simulink model "modelloTD_es1_sol2"  (R2021a)
settings: Solver=FixedStepDiscrete  StartTime=0.0  StopTime=10.0  FixedStep=0.001  RelTol=1e-3
values from neighbouring files (symbols this model uses):
  k = sym('k')    [fdt_es1.m]
  M1 = sym('M1')    [fdt_es1.m]
  M2 = sym('M2')    [fdt_es1.m]
undefined symbols (not defined in the file or in its folder): A1, A2, B1, B2, C1, C2
settings Model: Creator=User_LABORATORIO  LastModifiedBy=User_LABORATORIO

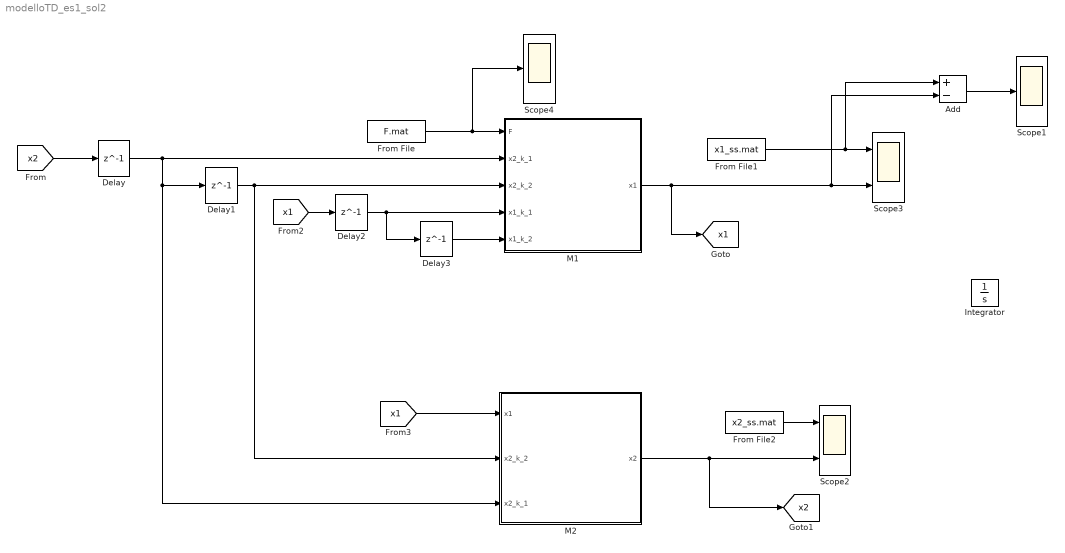
== system modelloTD_es1_sol2 ==
  Add : Sum  Inputs=+-
  Delay{,1..3} (4 alike) : Delay  DelayLength=1  InitialCondition=0
  From File : FromFile  FileName=F.mat  SampleTime=0
  From File1 : FromFile  FileName=x1_ss.mat  SampleTime=0
  From File2 : FromFile  FileName=x2_ss.mat  SampleTime=0
  Integrator : Integrator
  M1 : Subsystem
  M2 : Subsystem
  Scope1 : Scope
  Scope2 : Scope  NumInputPorts=2
  Scope3 : Scope  NumInputPorts=2
  Scope4 : Scope
  tag scope: x1=global, x2=global
  wires:
  Delay/1 -> M2/3(x2_k_1), Delay1/1, M1/2(x2_k_1)
  Add/1 -> Scope1/1
  M2/1(x2) -> [x2], Scope2/2
  [x1] -> M2/1(x1)
  From File1/1 -> Scope3/1, Add/1
  Delay3/1 -> M1/5(x1_k_2)
  [x1] -> Delay2/1
  Delay1/1 -> M2/2(x2_k_2), M1/3(x2_k_2)
  Delay2/1 -> Delay3/1, M1/4(x1_k_1)
  M1/1(x1) -> Scope3/2, Add/2, [x1]
  [x2] -> Delay/1
  From File/1 -> Scope4/1, M1/1(F)
  From File2/1 -> Scope2/1

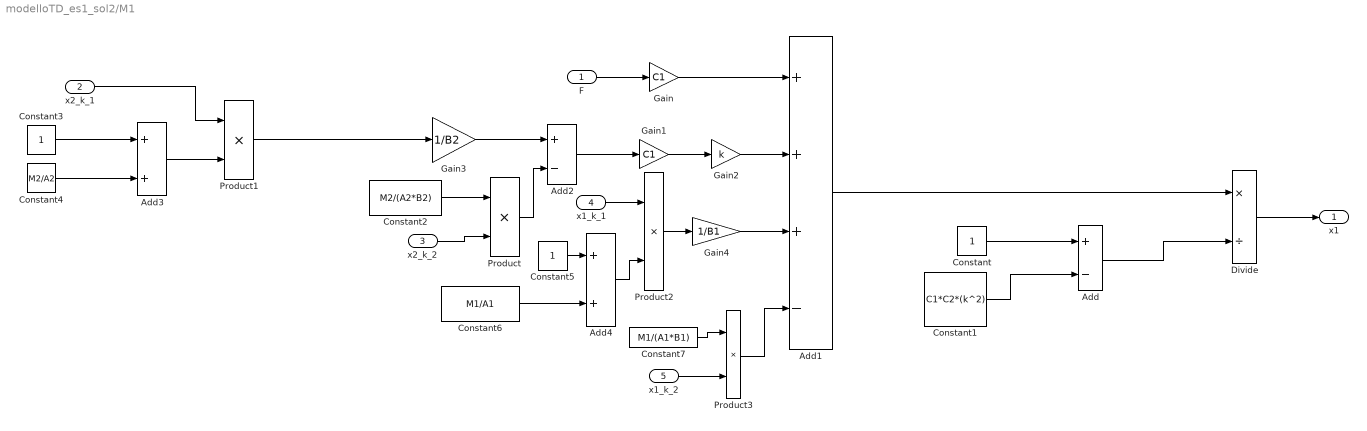
== system modelloTD_es1_sol2/M1 ==
  F : Inport
  x2_k_1 : Inport  Port=2
  x2_k_2 : Inport  Port=3
  x1_k_1 : Inport  Port=4
  x1_k_2 : Inport  Port=5
  Add : Sum  Inputs=+-
  Add1 : Sum  Inputs=+++-
  Add2 : Sum  Inputs=+-
  Add3 : Sum
  Add4 : Sum
  Constant : Constant
  Constant1 : Constant  Value=C1*C2*(k^2)
  Constant2 : Constant  Value=M2/(A2*B2)
  Constant3 : Constant
  Constant4 : Constant  Value=M2/A2
  Constant5 : Constant
  Constant6 : Constant  Value=M1/A1
  Constant7 : Constant  Value=M1/(A1*B1)
  Divide : Product  Inputs=*/
  Gain : Gain  Gain=C1
  Gain1 : Gain  Gain=C1
  Gain2 : Gain  Gain=k
  Gain3 : Gain  Gain=1/B2
  Gain4 : Gain  Gain=1/B1
  Product{,1..3} (4 alike) : Product
  x1 : Outport
  wires:
  Gain/1 -> Add1/1
  Constant3/1 -> Add3/1
  Product3/1 -> Add1/4
  Add/1 -> Divide/2
  Product/1 -> Add2/2
  x2_k_1/1 -> Product1/1
  F/1 -> Gain/1
  Constant/1 -> Add/1
  Divide/1 -> x1/1
  Constant1/1 -> Add/2
  Gain2/1 -> Add1/2
  Product1/1 -> Gain3/1
  Add1/1 -> Divide/1
  Constant4/1 -> Add3/2
  Gain1/1 -> Gain2/1
  Add3/1 -> Product1/2
  x1_k_2/1 -> Product3/2
  Add2/1 -> Gain1/1
  x2_k_2/1 -> Product/2
  Gain3/1 -> Add2/1
  x1_k_1/1 -> Product2/1
  Constant5/1 -> Add4/1
  Constant7/1 -> Product3/1
  Constant2/1 -> Product/1
  Add4/1 -> Product2/2
  Constant6/1 -> Add4/2
  Product2/1 -> Gain4/1
  Gain4/1 -> Add1/3

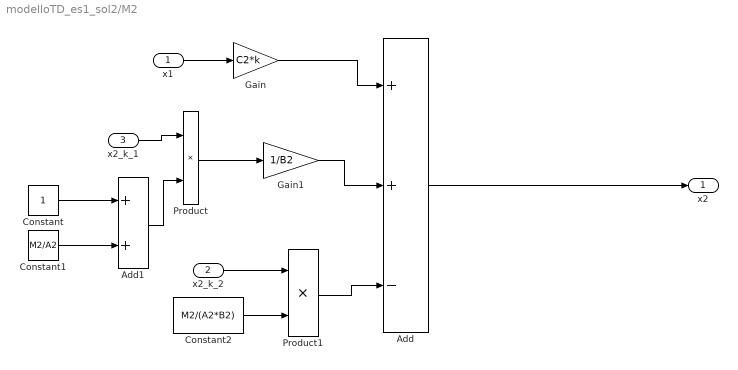
== system modelloTD_es1_sol2/M2 ==
  x1 : Inport
  x2_k_2 : Inport  Port=2
  x2_k_1 : Inport  Port=3
  Add : Sum  Inputs=++-
  Add1 : Sum
  Constant : Constant
  Constant1 : Constant  Value=M2/A2
  Constant2 : Constant  Value=M2/(A2*B2)
  Gain : Gain  Gain=C2*k
  Gain1 : Gain  Gain=1/B2
  Product : Product
  Product1 : Product
  x2 : Outport
  wires:
  Gain/1 -> Add/1
  Constant/1 -> Add1/1
  Add/1 -> x2/1
  x2_k_1/1 -> Product/1
  Constant1/1 -> Add1/2
  Constant2/1 -> Product1/2
  x2_k_2/1 -> Product1/1
  x1/1 -> Gain/1
  Product/1 -> Gain1/1
  Gain1/1 -> Add/2
  Add1/1 -> Product/2
  Product1/1 -> Add/3
